simulink model "BallAndBeam"  (R2018b)
settings: Solver=VariableStepAuto  StartTime=0.0  StopTime=ttotal  RelTol=1e-3
values from neighbouring files (symbols this model uses):
  tmuestra = 0.05    [IDDATA.m]    (also in Identificacion.m; PruebaMinCuadrados.m)
  var = 0.00001    (= 1e-05)    [Identificacion.m]    (also in PruebaMinCuadrados.m = 0.001)
undefined symbols (not defined in the file or in its folder): SimulBAB
settings Model: Creator=pablo  LastModifiedBy=pablo

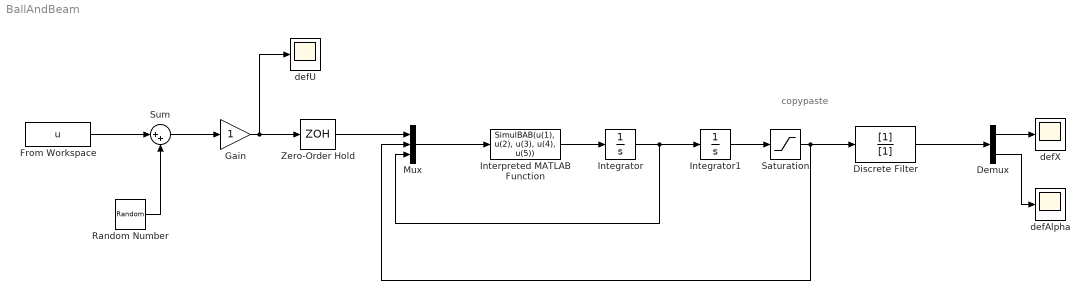
== system BallAndBeam ==
  note: copypaste
  Demux : Demux  Outputs=2
  Discrete Filter : DiscreteFilter  Denominator=[1]  SampleTime=tmuestra
  From Workspace : FromWorkspace  VariableName=u  SampleTime=tmuestra
  Gain : Gain
  Integrator : Integrator
  Integrator1 : Integrator
  Interpreted MATLAB Function : MATLABFcn  MATLABFcn=SimulBAB(u(1), u(2), u(3), u(4), u(5))  OutputDimensions=2
  Mux : Mux  Inputs=3
  Random Number : RandomNumber  Variance=var  Seed=354872  SampleTime=tmuestra
  Saturation : Saturate  UpperLimit=[0.4; 15*pi/180]  LowerLimit=-[0.4; 15*pi/180]
  Sum : Sum  Inputs=|++
  Zero-Order Hold : ZeroOrderHold  SampleTime=tmuestra
  "defAlpha " : Scope
  "defU " : Scope
  defX : Scope
  wires:
  From Workspace/1 -> Sum/1
  Random Number/1 -> Sum/2
  Gain/1 -> Zero-Order Hold/1, "defU "/1
  Sum/1 -> Gain/1
  Mux/1 -> Interpreted MATLAB Function/1
  Zero-Order Hold/1 -> Mux/1
  Integrator/1 -> Mux/3, Integrator1/1
  Interpreted MATLAB Function/1 -> Integrator/1
  Demux/2 -> "defAlpha "/1
  Demux/1 -> defX/1
  Integrator1/1 -> Saturation/1
  Saturation/1 -> Mux/2, Discrete Filter/1
  Discrete Filter/1 -> Demux/1
